simulink model "DoorLockCompositional"  (R2017b)
settings: Solver=FixedStepDiscrete  StartTime=0.0  StopTime=10.0  FixedStep=0.2  RelTol=1e-3
model workspace (MAT data in the model file):
  ContractValidatorBlocksMap = containers.Map
  ContractValidatorBlocksMap.serialization.keys = {'DoorLockCompositional/Lock/ControlSpec/validator', 'DoorLockCompositional/Lock/Keypad/CodeSpec/validator', 'DoorLockCompositional/Lock/KeypadSpec/validator', 'DoorLockCompositional/LockSpec/validator'}
  ContractValidatorBlocksMap.serialization.values{1}.block = 'DoorLockCompositional/Lock/ControlSpec/validator'
  ContractValidatorBlocksMap.serialization.values{1}.assumePorts = 0
  ContractValidatorBlocksMap.serialization.values{1}.guaranteePorts = 1
  ContractValidatorBlocksMap.serialization.values{1}.modeBlocksPorts = 0
  ContractValidatorBlocksMap.serialization.values{1}.portHandles.Inport = 2581.00549316
  ContractValidatorBlocksMap.serialization.values{1}.portHandles.Outport = 2582.00585938
  ContractValidatorBlocksMap.serialization.values{1}.portHandles.Enable = []
  ContractValidatorBlocksMap.serialization.values{1}.portHandles.Trigger = []
  ContractValidatorBlocksMap.serialization.values{1}.portHandles.State = []
  ContractValidatorBlocksMap.serialization.values{1}.portHandles.LConn = []
  ContractValidatorBlocksMap.serialization.values{1}.portHandles.RConn = []
  ContractValidatorBlocksMap.serialization.values{1}.portHandles.Ifaction = []
  ContractValidatorBlocksMap.serialization.values{1}.portHandles.Reset = []
  ContractValidatorBlocksMap.serialization.values{1}.portConnectivity(1).Type = '1'
  ContractValidatorBlocksMap.serialization.values{1}.portConnectivity(1).Position = [370 85]
  ContractValidatorBlocksMap.serialization.values{1}.portConnectivity(1).SrcBlock = 1865.00183105
  ContractValidatorBlocksMap.serialization.values{1}.portConnectivity(1).SrcPort = 0
  ContractValidatorBlocksMap.serialization.values{1}.portConnectivity(1).DstBlock = []
  ContractValidatorBlocksMap.serialization.values{1}.portConnectivity(1).DstPort = []
  ContractValidatorBlocksMap.serialization.values{1}.portConnectivity(2).Type = '1'
  ContractValidatorBlocksMap.serialization.values{1}.portConnectivity(2).Position = [500 85]
  ContractValidatorBlocksMap.serialization.values{1}.portConnectivity(2).SrcBlock = []
  ContractValidatorBlocksMap.serialization.values{1}.portConnectivity(2).SrcPort = []
  ContractValidatorBlocksMap.serialization.values{1}.portConnectivity(2).DstBlock = 1886.00170898
  ContractValidatorBlocksMap.serialization.values{1}.portConnectivity(2).DstPort = 0
  ContractValidatorBlocksMap.serialization.values{2}.block = 'DoorLockCompositional/Lock/Keypad/CodeSpec/validator'
  ContractValidatorBlocksMap.serialization.values{2}.assumePorts = 1
  ContractValidatorBlocksMap.serialization.values{2}.guaranteePorts = 1
  ContractValidatorBlocksMap.serialization.values{2}.modeBlocksPorts = 0
  ContractValidatorBlocksMap.serialization.values{2}.portHandles.Inport = [2578.0057373 2579.00598145]
  ContractValidatorBlocksMap.serialization.values{2}.portHandles.Outport = 2580.00585938
  ContractValidatorBlocksMap.serialization.values{2}.portHandles.Enable = []
  ContractValidatorBlocksMap.serialization.values{2}.portHandles.Trigger = []
  ContractValidatorBlocksMap.serialization.values{2}.portHandles.State = []
  ContractValidatorBlocksMap.serialization.values{2}.portHandles.LConn = []
  ContractValidatorBlocksMap.serialization.values{2}.portHandles.RConn = []
  ContractValidatorBlocksMap.serialization.values{2}.portHandles.Ifaction = []
  ContractValidatorBlocksMap.serialization.values{2}.portHandles.Reset = []
  ContractValidatorBlocksMap.serialization.values{2}.portConnectivity(1).Type = '1'
  ContractValidatorBlocksMap.serialization.values{2}.portConnectivity(1).Position = [385 50]
  ContractValidatorBlocksMap.serialization.values{2}.portConnectivity(1).SrcBlock = 1945.00256348
  ContractValidatorBlocksMap.serialization.values{2}.portConnectivity(1).SrcPort = 0
  ContractValidatorBlocksMap.serialization.values{2}.portConnectivity(1).DstBlock = []
  ContractValidatorBlocksMap.serialization.values{2}.portConnectivity(1).DstPort = []
  ContractValidatorBlocksMap.serialization.values{2}.portConnectivity(2).Type = '2'
  ContractValidatorBlocksMap.serialization.values{2}.portConnectivity(2).Position = [385 100]
  ContractValidatorBlocksMap.serialization.values{2}.portConnectivity(2).SrcBlock = 1959.00610352
  ContractValidatorBlocksMap.serialization.values{2}.portConnectivity(2).SrcPort = 0
  ContractValidatorBlocksMap.serialization.values{2}.portConnectivity(2).DstBlock = []
  ContractValidatorBlocksMap.serialization.values{2}.portConnectivity(2).DstPort = []
  ContractValidatorBlocksMap.serialization.values{2}.portConnectivity(3).Type = '1'
  ContractValidatorBlocksMap.serialization.values{2}.portConnectivity(3).Position = [475 75]
  ContractValidatorBlocksMap.serialization.values{2}.portConnectivity(3).SrcBlock = []
  ContractValidatorBlocksMap.serialization.values{2}.portConnectivity(3).SrcPort = []
  ContractValidatorBlocksMap.serialization.values{2}.portConnectivity(3).DstBlock = 1975.00280762
  ContractValidatorBlocksMap.serialization.values{2}.portConnectivity(3).DstPort = 0
  ContractValidatorBlocksMap.serialization.values{3}.block = 'DoorLockCompositional/Lock/KeypadSpec/validator'
  ContractValidatorBlocksMap.serialization.values{3}.assumePorts = 1
  ContractValidatorBlocksMap.serialization.values{3}.guaranteePorts = 5
  ContractValidatorBlocksMap.serialization.values{3}.modeBlocksPorts = 0
  ContractValidatorBlocksMap.serialization.values{3}.portHandles.Inport = [2571.00695801 2572.00598145 2573.0057373 2574.0057373 2575.0057373 2576.0057373]
  ContractValidatorBlocksMap.serialization.values{3}.portHandles.Outport = 2577.0057373
  ContractValidatorBlocksMap.serialization.values{3}.portHandles.Enable = []
  ContractValidatorBlocksMap.serialization.values{3}.portHandles.Trigger = []
  ContractValidatorBlocksMap.serialization.values{3}.portHandles.State = []
  ContractValidatorBlocksMap.serialization.values{3}.portHandles.LConn = []
  ContractValidatorBlocksMap.serialization.values{3}.portHandles.RConn = []
  ContractValidatorBlocksMap.serialization.values{3}.portHandles.Ifaction = []
  ContractValidatorBlocksMap.serialization.values{3}.portHandles.Reset = []
  ContractValidatorBlocksMap.serialization.values{3}.portConnectivity(1).Type = '1'
  ContractValidatorBlocksMap.serialization.values{3}.portConnectivity(1).Position = [365 -125]
  ContractValidatorBlocksMap.serialization.values{3}.portConnectivity(1).SrcBlock = 2195.00146484
  ContractValidatorBlocksMap.serialization.values{3}.portConnectivity(1).SrcPort = 0
  ContractValidatorBlocksMap.serialization.values{3}.portConnectivity(1).DstBlock = []
  ContractValidatorBlocksMap.serialization.values{3}.portConnectivity(1).DstPort = []
  ContractValidatorBlocksMap.serialization.values{3}.portConnectivity(2).Type = '2'
  ContractValidatorBlocksMap.serialization.values{3}.portConnectivity(2).Position = [365 -40]
  ContractValidatorBlocksMap.serialization.values{3}.portConnectivity(2).SrcBlock = 2229.00427246
  ContractValidatorBlocksMap.serialization.values{3}.portConnectivity(2).SrcPort = 0
  ContractValidatorBlocksMap.serialization.values{3}.portConnectivity(2).DstBlock = []
  ContractValidatorBlocksMap.serialization.values{3}.portConnectivity(2).DstPort = []
  ContractValidatorBlocksMap.serialization.values{3}.portConnectivity(3).Type = '3'
  ContractValidatorBlocksMap.serialization.values{3}.portConnectivity(3).Position = [365 45]
  ContractValidatorBlocksMap.serialization.values{3}.portConnectivity(3).SrcBlock = 2207.00341797
  ContractValidatorBlocksMap.serialization.values{3}.portConnectivity(3).SrcPort = 0
  ContractValidatorBlocksMap.serialization.values{3}.portConnectivity(3).DstBlock = []
  ContractValidatorBlocksMap.serialization.values{3}.portConnectivity(3).DstPort = []
  ContractValidatorBlocksMap.serialization.values{3}.portConnectivity(4).Type = '4'
  ContractValidatorBlocksMap.serialization.values{3}.portConnectivity(4).Position = [365 130]
  ContractValidatorBlocksMap.serialization.values{3}.portConnectivity(4).SrcBlock = 2257.01599121
  ContractValidatorBlocksMap.serialization.values{3}.portConnectivity(4).SrcPort = 0
  ContractValidatorBlocksMap.serialization.values{3}.portConnectivity(4).DstBlock = []
  ContractValidatorBlocksMap.serialization.values{3}.portConnectivity(4).DstPort = []
  ContractValidatorBlocksMap.serialization.values{3}.portConnectivity(5).Type = '5'
  ContractValidatorBlocksMap.serialization.values{3}.portConnectivity(5).Position = [365 215]
  ContractValidatorBlocksMap.serialization.values{3}.portConnectivity(5).SrcBlock = 2223.0057373
  ContractValidatorBlocksMap.serialization.values{3}.portConnectivity(5).SrcPort = 0
  ContractValidatorBlocksMap.serialization.values{3}.portConnectivity(5).DstBlock = []
  ContractValidatorBlocksMap.serialization.values{3}.portConnectivity(5).DstPort = []
  ContractValidatorBlocksMap.serialization.values{3}.portConnectivity(6).Type = '6'
  ContractValidatorBlocksMap.serialization.values{3}.portConnectivity(6).Position = [365 300]
  ContractValidatorBlocksMap.serialization.values{3}.portConnectivity(6).SrcBlock = 2247.00708008
  ContractValidatorBlocksMap.serialization.values{3}.portConnectivity(6).SrcPort = 0
  ContractValidatorBlocksMap.serialization.values{3}.portConnectivity(6).DstBlock = []
  ContractValidatorBlocksMap.serialization.values{3}.portConnectivity(6).DstPort = []
  ContractValidatorBlocksMap.serialization.values{3}.portConnectivity(7).Type = '1'
  ContractValidatorBlocksMap.serialization.values{3}.portConnectivity(7).Position = [500 90]
  ContractValidatorBlocksMap.serialization.values{3}.portConnectivity(7).SrcBlock = []
  ContractValidatorBlocksMap.serialization.values{3}.portConnectivity(7).SrcPort = []
  ContractValidatorBlocksMap.serialization.values{3}.portConnectivity(7).DstBlock = [2282.00183105 2194.00244141]
  ContractValidatorBlocksMap.serialization.values{3}.portConnectivity(7).DstPort = [0 0]
  ContractValidatorBlocksMap.serialization.values{4}.block = 'DoorLockCompositional/LockSpec/validator'
  ContractValidatorBlocksMap.serialization.values{4}.assumePorts = 1
  ContractValidatorBlocksMap.serialization.values{4}.guaranteePorts = 2
  ContractValidatorBlocksMap.serialization.values{4}.modeBlocksPorts = 0
  ContractValidatorBlocksMap.serialization.values{4}.portHandles.Inport = [2583.00549316 2584.00549316 2585.00585938]
  ContractValidatorBlocksMap.serialization.values{4}.portHandles.Outport = 2586.00549316
  ContractValidatorBlocksMap.serialization.values{4}.portHandles.Enable = []
  ContractValidatorBlocksMap.serialization.values{4}.portHandles.Trigger = []
  ContractValidatorBlocksMap.serialization.values{4}.portHandles.State = []
  ContractValidatorBlocksMap.serialization.values{4}.portHandles.LConn = []
  ContractValidatorBlocksMap.serialization.values{4}.portHandles.RConn = []
  ContractValidatorBlocksMap.serialization.values{4}.portHandles.Ifaction = []
  ContractValidatorBlocksMap.serialization.values{4}.portHandles.Reset = []
  ContractValidatorBlocksMap.serialization.values{4}.portConnectivity(1).Type = '1'
  ContractValidatorBlocksMap.serialization.values{4}.portConnectivity(1).Position = [445 -95]
  ContractValidatorBlocksMap.serialization.values{4}.portConnectivity(1).SrcBlock = 2413.00170898
  ContractValidatorBlocksMap.serialization.values{4}.portConnectivity(1).SrcPort = 0
  ContractValidatorBlocksMap.serialization.values{4}.portConnectivity(1).DstBlock = []
  ContractValidatorBlocksMap.serialization.values{4}.portConnectivity(1).DstPort = []
  ContractValidatorBlocksMap.serialization.values{4}.portConnectivity(2).Type = '2'
  ContractValidatorBlocksMap.serialization.values{4}.portConnectivity(2).Position = [445 75]
  ContractValidatorBlocksMap.serialization.values{4}.portConnectivity(2).SrcBlock = 2425.00341797
  ContractValidatorBlocksMap.serialization.values{4}.portConnectivity(2).SrcPort = 0
  ContractValidatorBlocksMap.serialization.values{4}.portConnectivity(2).DstBlock = []
  ContractValidatorBlocksMap.serialization.values{4}.portConnectivity(2).DstPort = []
  ContractValidatorBlocksMap.serialization.values{4}.portConnectivity(3).Type = '3'
  ContractValidatorBlocksMap.serialization.values{4}.portConnectivity(3).Position = [445 245]
  ContractValidatorBlocksMap.serialization.values{4}.portConnectivity(3).SrcBlock = 2431.00341797
  ContractValidatorBlocksMap.serialization.values{4}.portConnectivity(3).SrcPort = 0
  ContractValidatorBlocksMap.serialization.values{4}.portConnectivity(3).DstBlock = []
  ContractValidatorBlocksMap.serialization.values{4}.portConnectivity(3).DstPort = []
  ContractValidatorBlocksMap.serialization.values{4}.portConnectivity(4).Type = '1'
  ContractValidatorBlocksMap.serialization.values{4}.portConnectivity(4).Position = [580 75]
  ContractValidatorBlocksMap.serialization.values{4}.portConnectivity(4).SrcBlock = []
  ContractValidatorBlocksMap.serialization.values{4}.portConnectivity(4).SrcPort = []
  ContractValidatorBlocksMap.serialization.values{4}.portConnectivity(4).DstBlock = [2539.00231934 2411.00268555]
  ContractValidatorBlocksMap.serialization.values{4}.portConnectivity(4).DstPort = [0 0]
  ContractValidatorBlocksMap.serialization.uniformity = 0
  ContractValidatorBlocksMap.serialization.keyType = 'char'
  ContractValidatorBlocksMap.serialization.valueType = 'any'
undefined symbols (not defined in the file): contractAfterSimulation, ContractAssumeBlock, contractBeforeSimulation, ContractBlock, ContractGuaranteeBlock, ContractValidatorBlock, saveValidatorParameters
libraries: simulink x17, Kind x15
settings Model: Creator=mahgoubyahia  LastModifiedBy=hbourbou
settings OptimizationCC: LifeSpan=inf
settings DebuggingCC: SFExecutionAtInitializationDiag=none
settings HardwareCC: ProdBitPerSizeT=32  ProdBitPerPtrDiffT=32  ProdWordSize=32  ProdHWDeviceType=Specified
settings CodeAppCC: StateflowObjectComments=on

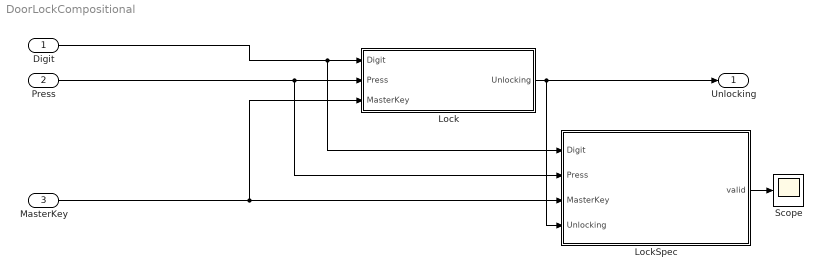
== system DoorLockCompositional ==
  Digit : Inport  OutDataTypeStr=int8
  Press : Inport  Port=2  OutDataTypeStr=boolean
  MasterKey : Inport  Port=3  OutDataTypeStr=boolean
  Lock : Subsystem
  LockSpec : Subsystem  mask(ContractBlock){ContractBlockType=ContractBlock}
      mask DialogControl DescTextVar Prompt: Contract block
      mask Display:
      | text(0.5, 0.5, '{\bf\fontsize{20}Contract}', 'hor', 'center', 'texmode','on');
      | blocks = find_system(gcb, 'LookUnderMasks','all', 'SearchDepth',1,'BlockType','Inport');
      | for i = 1 : length(blocks)
      |     blockName = get_param(blocks(i), 'Name');
      |     [path, blockName] = fileparts(char(blockName));
      |     port_label('input', i, blockName);
      | end
      | 
      | blocks = find_system(gcb, 'LookUnderMasks','all', 'SearchDepth',1,'BlockType','Outport');
      | for i = 1 : length(blocks)
      |     blockName = get_param(blocks(i), 'Name');
      |     [path, blockName] = fileparts(char(blockName));
      |     port_label('output', i, blockName);
      | end
  Scope : Scope
  Unlocking : Outport  OutDataTypeStr=boolean
  wires:
  Digit/1 -> LockSpec/1(Digit), Lock/1(Digit)
  Press/1 -> LockSpec/2(Press), Lock/2(Press)
  MasterKey/1 -> Lock/3(MasterKey), LockSpec/3(MasterKey)
  Lock/1(Unlocking) -> LockSpec/4(Unlocking), Unlocking/1
  LockSpec/1(valid) -> Scope/1

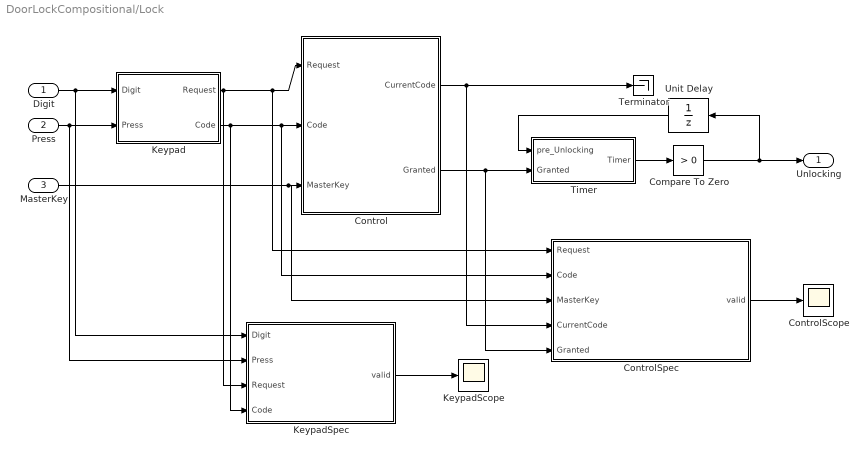
== system DoorLockCompositional/Lock ==
  Digit : Inport  OutDataTypeStr=int8
  Press : Inport  Port=2  OutDataTypeStr=boolean
  MasterKey : Inport  Port=3  OutDataTypeStr=boolean
  Compare To Zero : simulink/Logic and Bit Operations/Compare To Zero  relop=>  OutDataTypeStr=boolean
  Control : Subsystem
  ControlScope : Scope
  ControlSpec : Subsystem  AncestorBlock=Kind/contract  mask(ContractBlock){ContractBlockType=ContractBlock}
      mask init:
      | set_param(gcb, 'LinkStatus', 'inactive');
      mask DialogControl DescTextVar Prompt: Contract block
      mask Display:
      | text(0.5, 0.5, '{\bf\fontsize{20}Contract}', 'hor', 'center', 'texmode','on');
      | blocks = find_system(gcb, 'LookUnderMasks','all', 'SearchDepth',1,'BlockType','Inport');
      | for i = 1 : length(blocks)
      |     blockName = get_param(blocks(i), 'Name');
      |     [path, blockName] = fileparts(char(blockName));
      |     port_label('input', i, blockName);
      | end
      | 
      | blocks = find_system(gcb, 'LookUnderMasks','all', 'SearchDepth',1,'BlockType','Outport');
      | for i = 1 : length(blocks)
      |     blockName = get_param(blocks(i), 'Name');
      |     [path, blockName] = fileparts(char(blockName));
      |     port_label('output', i, blockName);
      | end
  Keypad : Subsystem
  KeypadScope : Scope
  KeypadSpec : Subsystem  mask(ContractBlock){ContractBlockType=ContractBlock}
      mask init:
      | set_param(gcb, 'LinkStatus', 'none');
      mask DialogControl DescTextVar Prompt: Contract block
      mask Display:
      | text(0.5, 0.5, '{\bf\fontsize{20}Contract}', 'hor', 'center', 'texmode','on');
      | blocks = find_system(gcb, 'LookUnderMasks','all', 'SearchDepth',1,'BlockType','Inport');
      | for i = 1 : length(blocks)
      |     blockName = get_param(blocks(i), 'Name');
      |     [path, blockName] = fileparts(char(blockName));
      |     port_label('input', i, blockName);
      | end
      | 
      | blocks = find_system(gcb, 'LookUnderMasks','all', 'SearchDepth',1,'BlockType','Outport');
      | for i = 1 : length(blocks)
      |     blockName = get_param(blocks(i), 'Name');
      |     [path, blockName] = fileparts(char(blockName));
      |     port_label('output', i, blockName);
      | end
  Terminator : Terminator
  Timer : Subsystem
  Unit Delay : UnitDelay  SampleTime=-1
  Unlocking : Outport  OutDataTypeStr=boolean
  wires:
  Control/1(CurrentCode) -> ControlSpec/4(CurrentCode), Terminator/1
  Keypad/2(Code) -> KeypadSpec/4(Code), Control/2(Code), ControlSpec/2(Code)
  Keypad/1(Request) -> KeypadSpec/3(Request), Control/1(Request), ControlSpec/1(Request)
  MasterKey/1 -> ControlSpec/3(MasterKey), Control/3(MasterKey)
  Timer/1(Timer) -> Compare To Zero/1
  Compare To Zero/1 -> Unlocking/1, Unit Delay/1
  Press/1 -> KeypadSpec/2(Press), Keypad/2(Press)
  Digit/1 -> KeypadSpec/1(Digit), Keypad/1(Digit)
  Control/2(Granted) -> ControlSpec/5(Granted), Timer/2(Granted)
  ControlSpec/1(valid) -> ControlScope/1
  KeypadSpec/1(valid) -> KeypadScope/1
  Unit Delay/1 -> Timer/1(pre_Unlocking)

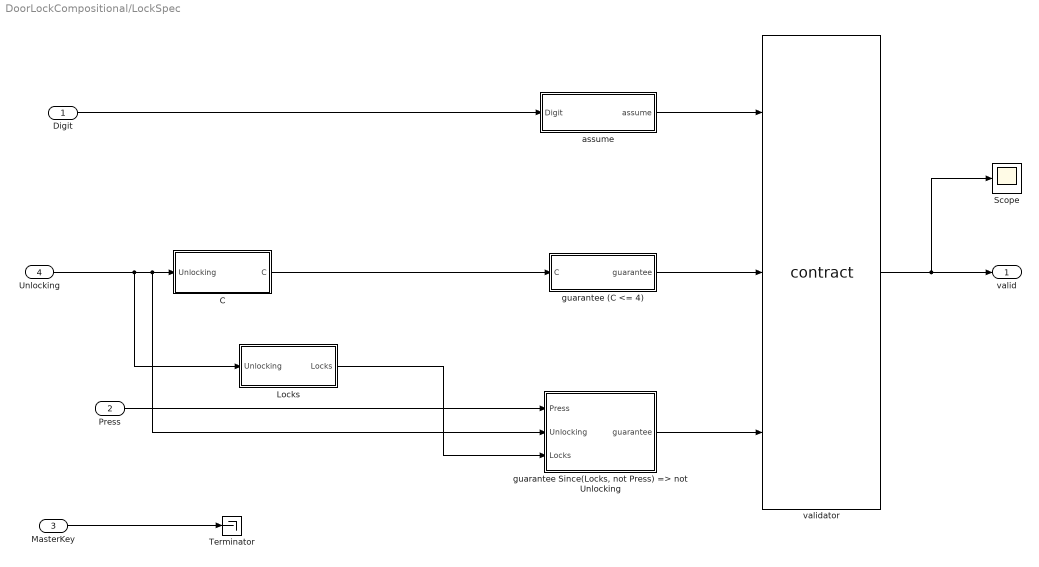
== system DoorLockCompositional/LockSpec ==
  Digit : Inport
  Press : Inport  Port=2  OutDataTypeStr=boolean
  MasterKey : Inport  Port=3  OutDataTypeStr=boolean
  Unlocking : Inport  Port=4  OutDataTypeStr=boolean
  C : Subsystem
  Locks : Subsystem
  Scope : Scope
  Terminator : Terminator
  assume : Subsystem  AncestorBlock=Kind/assume  mask(ContractAssumeBlock){ContractBlockType=ContractAssumeBlock}
      mask DialogControl DescTextVar Prompt: Assume block
  guarantee (C <= 4) : Subsystem  AncestorBlock=Kind/guarantee  mask(ContractGuaranteeBlock){ContractBlockType=ContractGuaranteeBlock}
      mask DialogControl DescTextVar Prompt: Guarantee block
  "guarantee Since(Locks, not Press) => not Unlocking" : Subsystem  AncestorBlock=Kind/guarantee  mask(ContractGuaranteeBlock){ContractBlockType=ContractGuaranteeBlock}
      mask DialogControl DescTextVar Prompt: Guarantee block
  validator : M-S-Function  LoadFcn=saveValidatorParameters(gcb);  InitFcn=contractBeforeSimulation();  StopFcn=contractAfterSimulation();  FunctionName=contract  mask(ContractValidatorBlock){assumePorts=1, guaranteePorts=2, modePorts=0, ContractBlockType=ContractValidatorBlock, createInportsCheckbox=off}
      mask prompts: assumePorts "Assume ports     :"; guaranteePorts "Guarantee ports :"; modePorts "Mode ports        :"; createInportsCheckbox "Create inports and connect them automatically"
      mask init:
      | set_param(gcb,'LinkStatus','none');
      | contract_callback('inputs_callback',gcb);
      mask DialogControl DescTextVar Prompt: The validator block implements the following logic: <br> <br> <b>Sofar</b>(assume<sub>1</sub> <b>&#8743;</b> assume<sub>2</sub> <b>&#8743;</b> ... assume<sub>k</sub>) <b>&rarr;</b> (guarantee<sub>1</sub> <b>&#8743;</b> guarantee<sub>2</sub> <b>&#8743;</b> ... guarantee<sub>m</sub> <b>&#8743;</b>  mode<sub>1</sub> <b>&#8743;</b> mode<sub>2</sub> <b>&#8743;</b> ... <b>&#8743;</b> mode<sub>n</sub> )<br> where mode<sub>i</sub> = require<sub>i</sub> <b>&rarr;</b> ensure<sub>i</sub>
      mask Display:
      | color('black');
      | port_label('input',1,'assume');
      | port_label('input',2,'guarantee');
      | port_label('input',3,'guarantee');
      | port_label('output',1,'valid');
  valid : Outport
  wires:
  validator/1 -> Scope/1, valid/1
  assume/1(assume) -> validator/1
  guarantee (C <= 4)/1(guarantee) -> validator/2
  "guarantee Since(Locks, not Press) => not Unlocking"/1(guarantee) -> validator/3
  Digit/1 -> assume/1(Digit)
  Press/1 -> "guarantee Since(Locks, not Press) => not Unlocking"/1(Press)
  Unlocking/1 -> Locks/1(Unlocking), "guarantee Since(Locks, not Press) => not Unlocking"/2(Unlocking), C/1(Unlocking)
  C/1(C) -> guarantee (C <= 4)/1(C)
  MasterKey/1 -> Terminator/1
  Locks/1(Locks) -> "guarantee Since(Locks, not Press) => not Unlocking"/3(Locks)

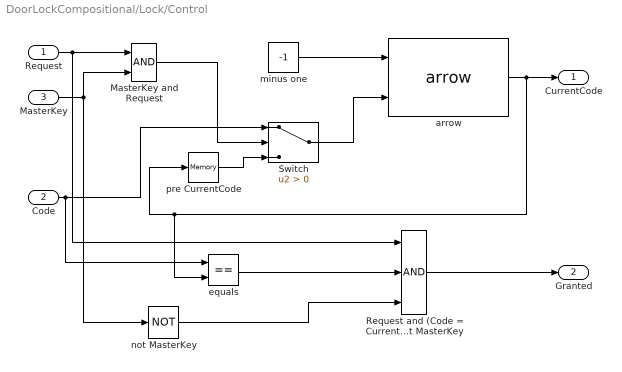
== system DoorLockCompositional/Lock/Control ==
  Request : Inport  OutDataTypeStr=boolean
  Code : Inport  Port=2  OutDataTypeStr=int32
  MasterKey : Inport  Port=3  OutDataTypeStr=boolean
  MasterKey and Request : Logic  IconShape=distinctive  AllPortsSameDT=off  OutDataTypeStr=boolean
  Request and (Code = CurrentCode) and not MasterKey : Logic  Inputs=3  IconShape=distinctive  AllPortsSameDT=off  OutDataTypeStr=boolean
  Switch : Switch  Criteria=u2 > Threshold
  arrow : Kind/arrow  LustreOperatorBlock=ArrowOperator
  equals : RelationalOperator  Operator===  OutDataTypeStr=boolean  RndMeth=Nearest
  minus one : Constant  Value=-1  OutDataTypeStr=int32
  "not MasterKey " : Logic  Operator=NOT  IconShape=distinctive  AllPortsSameDT=off  OutDataTypeStr=boolean
  pre CurrentCode : Memory
  CurrentCode : Outport  OutDataTypeStr=int32
  Granted : Outport  Port=2  OutDataTypeStr=boolean
  wires:
  arrow/1 -> equals/2, pre CurrentCode/1, CurrentCode/1
  minus one/1 -> arrow/1
  Request/1 -> MasterKey and Request/1, Request and (Code = CurrentCode) and not MasterKey/1
  MasterKey/1 -> "not MasterKey "/1, MasterKey and Request/2
  MasterKey and Request/1 -> Switch/2
  Code/1 -> equals/1, Switch/1
  pre CurrentCode/1 -> Switch/3
  Switch/1 -> arrow/2
  equals/1 -> Request and (Code = CurrentCode) and not MasterKey/2
  "not MasterKey "/1 -> Request and (Code = CurrentCode) and not MasterKey/3
  Request and (Code = CurrentCode) and not MasterKey/1 -> Granted/1

== system DoorLockCompositional/Lock/ControlSpec ==
  Request : Inport  OutDataTypeStr=boolean
  Code : Inport  Port=2  OutDataTypeStr=int32
  MasterKey : Inport  Port=3  OutDataTypeStr=boolean
  CurrentCode : Inport  Port=4  OutDataTypeStr=int32
  Granted : Inport  Port=5  OutDataTypeStr=boolean
  guarantee true : Subsystem  mask(ContractGuaranteeBlock){ContractBlockType=ContractGuaranteeBlock}
      mask init:
      | set_param(gcb, 'LinkStatus', 'none');
      mask DialogControl DescTextVar Prompt: Guarantee block
  validator : M-S-Function  LoadFcn=saveValidatorParameters(gcb);  InitFcn=contractBeforeSimulation();  StopFcn=contractAfterSimulation();  FunctionName=contract  mask(ContractValidatorBlock){assumePorts=0, guaranteePorts=1, modePorts=0, ContractBlockType=ContractValidatorBlock, createInportsCheckbox=off}
      mask prompts: assumePorts "Assume ports     :"; guaranteePorts "Guarantee ports :"; modePorts "Mode ports        :"; createInportsCheckbox "Create inports and connect them automatically"
      mask init:
      | set_param(gcb,'LinkStatus','none');
      | contract_callback('inputs_callback',gcb);
      mask DialogControl DescTextVar Prompt: The validator block implements the following logic: <br> <br> <b>Sofar</b>(assume<sub>1</sub> <b>&#8743;</b> assume<sub>2</sub> <b>&#8743;</b> ... assume<sub>k</sub>) <b>&rarr;</b> (guarantee<sub>1</sub> <b>&#8743;</b> guarantee<sub>2</sub> <b>&#8743;</b> ... guarantee<sub>m</sub> <b>&#8743;</b>  mode<sub>1</sub> <b>&#8743;</b> mode<sub>2</sub> <b>&#8743;</b> ... <b>&#8743;</b> mode<sub>n</sub> )<br> where mode<sub>i</sub> = require<sub>i</sub> <b>&rarr;</b> ensure<sub>i</sub>
      mask Display:
      | color('black');
      | port_label('input',1,'guarantee');
      | port_label('output',1,'valid');
  valid : Outport
  wires:
  validator/1 -> valid/1
  guarantee true/1(guarantee) -> validator/1
  Request/1 -> guarantee true/1(Request)
  Code/1 -> guarantee true/2(Code)
  MasterKey/1 -> guarantee true/3(MasterKey)
  CurrentCode/1 -> guarantee true/4(CurrentCode)
  Granted/1 -> guarantee true/5(Granted)

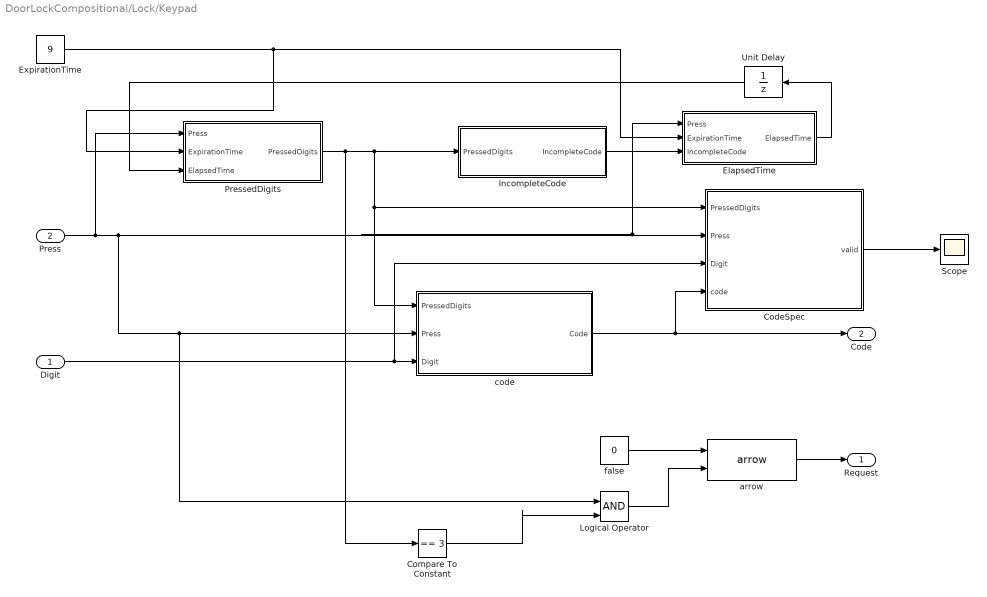
== system DoorLockCompositional/Lock/Keypad ==
  Digit : Inport
  Press : Inport  Port=2  OutDataTypeStr=boolean
  CodeSpec : Subsystem  mask(ContractBlock){ContractBlockType=ContractBlock}
      mask init:
      | set_param(gcb, 'LinkStatus', 'none');
      settings: CopyFcn=set_param(gcb, 'LinkStatus', 'none');
      mask DialogControl DescTextVar Prompt: Contract block
      mask Display:
      | text(0.5, 0.5, '{\bf\fontsize{20}Contract}', 'hor', 'center', 'texmode','on');
      | blocks = find_system(gcb, 'LookUnderMasks','all', 'SearchDepth',1,'BlockType','Inport');
      | for i = 1 : length(blocks)
      |     blockName = get_param(blocks(i), 'Name');
      |     [path, blockName] = fileparts(char(blockName));
      |     port_label('input', i, blockName);
      | end
      | 
      | blocks = find_system(gcb, 'LookUnderMasks','all', 'SearchDepth',1,'BlockType','Outport');
      | for i = 1 : length(blocks)
      |     blockName = get_param(blocks(i), 'Name');
      |     [path, blockName] = fileparts(char(blockName));
      |     port_label('output', i, blockName);
      | end
  Compare To Constant : simulink/Logic and Bit Operations/Compare To Constant  relop===  const=3  OutDataTypeStr=boolean
  ElapsedTime : Subsystem
  ExpirationTime : Constant  Value=9  OutDataTypeStr=int32
  IncompleteCode : Subsystem
  Logical Operator : Logic  IconShape=distinctive  AllPortsSameDT=off  OutDataTypeStr=boolean
  PressedDigits : Subsystem
  Scope : Scope
  Unit Delay : UnitDelay  SampleTime=-1
  arrow : Kind/arrow  LustreOperatorBlock=ArrowOperator
  code : Subsystem
  false : Constant  Value=0  OutDataTypeStr=boolean
  Request : Outport  OutDataTypeStr=boolean
  Code : Outport  Port=2  OutDataTypeStr=int32
  wires:
  PressedDigits/1(PressedDigits) -> Compare To Constant/1, code/1(PressedDigits), CodeSpec/1(PressedDigits), IncompleteCode/1(PressedDigits)
  Press/1 -> PressedDigits/1(Press), Logical Operator/1, code/2(Press), CodeSpec/2(Press), ElapsedTime/1(Press)
  ExpirationTime/1 -> ElapsedTime/2(ExpirationTime), PressedDigits/2(ExpirationTime)
  IncompleteCode/1(IncompleteCode) -> ElapsedTime/3(IncompleteCode)
  ElapsedTime/1(ElapsedTime) -> Unit Delay/1
  Digit/1 -> CodeSpec/3(Digit), code/3(Digit)
  code/1(Code) -> CodeSpec/4(code), Code/1
  arrow/1 -> Request/1
  false/1 -> arrow/1
  Logical Operator/1 -> arrow/2
  Compare To Constant/1 -> Logical Operator/2
  CodeSpec/1(valid) -> Scope/1
  Unit Delay/1 -> PressedDigits/3(ElapsedTime)

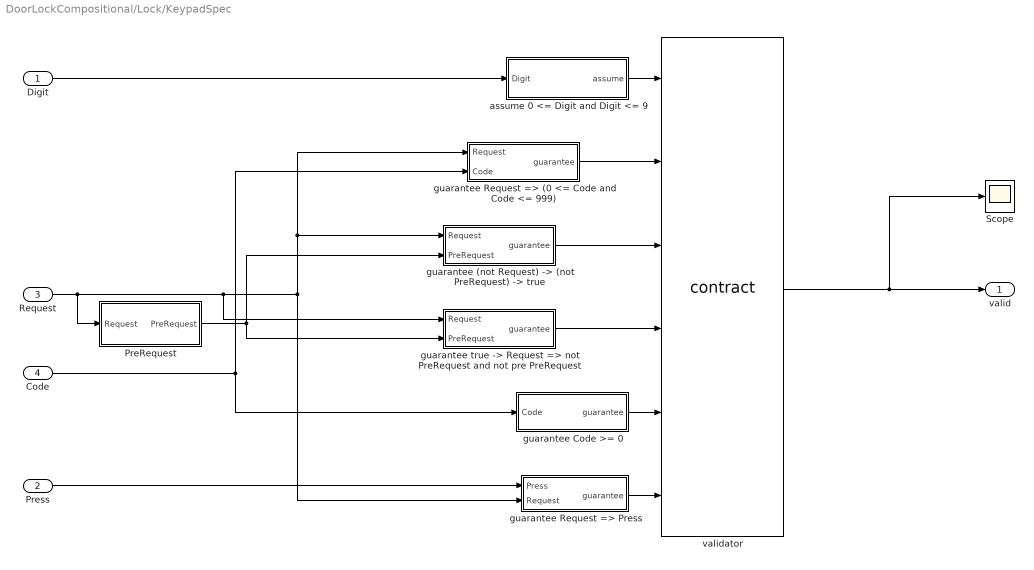
== system DoorLockCompositional/Lock/KeypadSpec ==
  Digit : Inport
  Press : Inport  Port=2  OutDataTypeStr=boolean
  Request : Inport  Port=3  OutDataTypeStr=boolean
  Code : Inport  Port=4  OutDataTypeStr=int32
  PreRequest : Subsystem
  Scope : Scope
  assume 0 <= Digit and Digit <= 9 : Subsystem  mask(ContractAssumeBlock){ContractBlockType=ContractAssumeBlock}
      mask init:
      | set_param(gcb, 'LinkStatus', 'none');
      mask DialogControl DescTextVar Prompt: Assume block
  "guarantee (not Request) -> (not PreRequest) -> true" : Subsystem  mask(ContractGuaranteeBlock){ContractBlockType=ContractGuaranteeBlock}
      mask init:
      | set_param(gcb, 'LinkStatus', 'none');
      mask DialogControl DescTextVar Prompt: Guarantee block
  guarantee Code >= 0 : Subsystem  mask(ContractGuaranteeBlock){ContractBlockType=ContractGuaranteeBlock}
      mask init:
      | set_param(gcb, 'LinkStatus', 'none');
      mask DialogControl DescTextVar Prompt: Guarantee block
  guarantee Request => (0 <= Code and Code <= 999) : Subsystem  mask(ContractGuaranteeBlock){ContractBlockType=ContractGuaranteeBlock}
      mask init:
      | set_param(gcb, 'LinkStatus', 'none');
      mask DialogControl DescTextVar Prompt: Guarantee block
  guarantee Request => Press : Subsystem  mask(ContractGuaranteeBlock){ContractBlockType=ContractGuaranteeBlock}
      mask init:
      | set_param(gcb, 'LinkStatus', 'none');
      mask DialogControl DescTextVar Prompt: Guarantee block
  "guarantee true -> Request => not PreRequest and not pre PreRequest" : Subsystem  mask(ContractGuaranteeBlock){ContractBlockType=ContractGuaranteeBlock}
      mask init:
      | set_param(gcb, 'LinkStatus', 'none');
      mask DialogControl DescTextVar Prompt: Guarantee block
  validator : M-S-Function  LoadFcn=saveValidatorParameters(gcb);  InitFcn=contractBeforeSimulation();  StopFcn=contractAfterSimulation();  FunctionName=contract  mask(ContractValidatorBlock){assumePorts=1, guaranteePorts=5, modePorts=0, ContractBlockType=ContractValidatorBlock, createInportsCheckbox=off}
      mask prompts: assumePorts "Assume ports     :"; guaranteePorts "Guarantee ports :"; modePorts "Mode ports        :"; createInportsCheckbox "Create inports and connect them automatically"
      mask init:
      | set_param(gcb,'LinkStatus','none');
      | contract_callback('inputs_callback',gcb);
      mask DialogControl DescTextVar Prompt: The validator block implements the following logic: <br> <br> <b>Sofar</b>(assume<sub>1</sub> <b>&#8743;</b> assume<sub>2</sub> <b>&#8743;</b> ... assume<sub>k</sub>) <b>&rarr;</b> (guarantee<sub>1</sub> <b>&#8743;</b> guarantee<sub>2</sub> <b>&#8743;</b> ... guarantee<sub>m</sub> <b>&#8743;</b>  mode<sub>1</sub> <b>&#8743;</b> mode<sub>2</sub> <b>&#8743;</b> ... <b>&#8743;</b> mode<sub>n</sub> )<br> where mode<sub>i</sub> = require<sub>i</sub> <b>&rarr;</b> ensure<sub>i</sub>
      mask Display:
      | color('black');
      | port_label('input',1,'assume');
      | port_label('input',2,'guarantee');
      | port_label('input',3,'guarantee');
      | port_label('input',4,'guarantee');
      | port_label('input',5,'guarantee');
      | port_label('input',6,'guarantee');
      | port_label('output',1,'valid');
  valid : Outport
  wires:
  validator/1 -> Scope/1, valid/1
  assume 0 <= Digit and Digit <= 9/1(assume) -> validator/1
  guarantee Request => (0 <= Code and Code <= 999)/1(guarantee) -> validator/2
  "guarantee (not Request) -> (not PreRequest) -> true"/1(guarantee) -> validator/3
  guarantee Code >= 0/1(guarantee) -> validator/5
  guarantee Request => Press/1(guarantee) -> validator/6
  Digit/1 -> assume 0 <= Digit and Digit <= 9/1(Digit)
  Press/1 -> guarantee Request => Press/1(Press)
  Request/1 -> PreRequest/1(Request), "guarantee true -> Request => not PreRequest and not pre PreRequest"/1(Request), guarantee Request => Press/2(Request), guarantee Request => (0 <= Code and Code <= 999)/1(Request), "guarantee (not Request) -> (not PreRequest) -> true"/1(Request)
  Code/1 -> guarantee Code >= 0/1(Code), guarantee Request => (0 <= Code and Code <= 999)/2(Code)
  PreRequest/1(PreRequest) -> "guarantee true -> Request => not PreRequest and not pre PreRequest"/2(PreRequest), "guarantee (not Request) -> (not PreRequest) -> true"/2(PreRequest)
  "guarantee true -> Request => not PreRequest and not pre PreRequest"/1(guarantee) -> validator/4

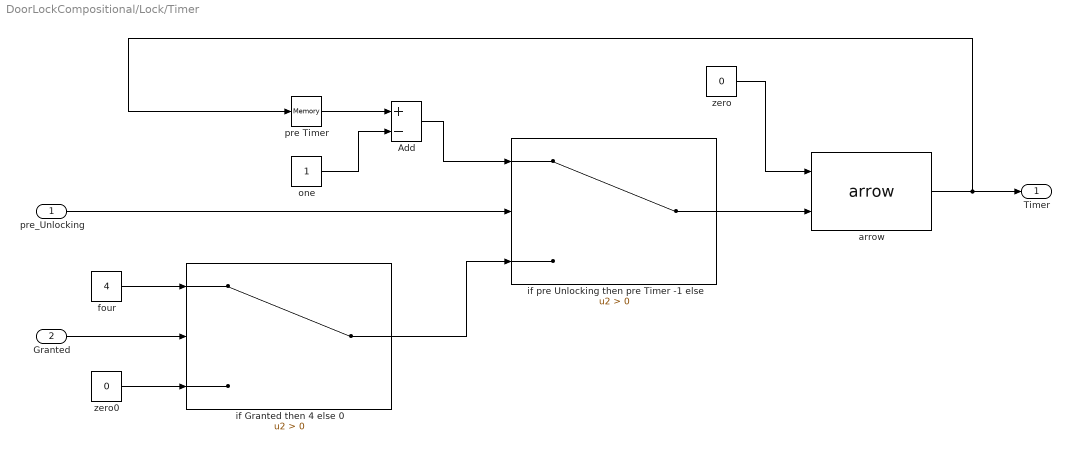
== system DoorLockCompositional/Lock/Timer ==
  pre_Unlocking : Inport  OutDataTypeStr=boolean
  Granted : Inport  Port=2  OutDataTypeStr=boolean
  Add : Sum  Inputs=+-
  arrow : Kind/arrow  LustreOperatorBlock=ArrowOperator
  four : Constant  Value=4  OutDataTypeStr=int32
  if Granted then 4 else 0 : Switch  Criteria=u2 > Threshold
  if pre Unlocking then pre Timer -1 else : Switch  Criteria=u2 > Threshold
  one : Constant  OutDataTypeStr=int32
  pre Timer : Memory
  zero : Constant  Value=0  OutDataTypeStr=int32
  zero0 : Constant  Value=0  OutDataTypeStr=int32
  Timer : Outport
  wires:
  zero/1 -> arrow/1
  arrow/1 -> pre Timer/1, Timer/1
  pre_Unlocking/1 -> if pre Unlocking then pre Timer -1 else/2
  pre Timer/1 -> Add/1
  one/1 -> Add/2
  Add/1 -> if pre Unlocking then pre Timer -1 else/1
  Granted/1 -> if Granted then 4 else 0/2
  four/1 -> if Granted then 4 else 0/1
  zero0/1 -> if Granted then 4 else 0/3
  if Granted then 4 else 0/1 -> if pre Unlocking then pre Timer -1 else/3
  if pre Unlocking then pre Timer -1 else/1 -> arrow/2

== system DoorLockCompositional/LockSpec/C ==
  Unlocking : Inport  OutDataTypeStr=boolean
  Add : Sum
  Switch : Switch  Criteria=u2 > Threshold
  arrow : Kind/arrow  LustreOperatorBlock=ArrowOperator
  one : Constant  OutDataTypeStr=int32
  one1 : Constant  OutDataTypeStr=int32
  pre C : Memory
  zero : Constant  Value=0  OutDataTypeStr=int32
  C : Outport  OutDataTypeStr=int32
  wires:
  Unlocking/1 -> Switch/2
  one/1 -> arrow/1
  one1/1 -> Add/2
  pre C/1 -> Add/1
  Add/1 -> arrow/2
  arrow/1 -> Switch/1
  Switch/1 -> pre C/1, C/1
  zero/1 -> Switch/3

== system DoorLockCompositional/LockSpec/Locks ==
  Unlocking : Inport  OutDataTypeStr=boolean
  and : Logic  IconShape=distinctive  AllPortsSameDT=off  OutDataTypeStr=boolean
  arrow : Kind/arrow  LustreOperatorBlock=ArrowOperator
  false : Constant  Value=0  OutDataTypeStr=boolean
  not Unlocking : Logic  Operator=NOT  IconShape=distinctive  AllPortsSameDT=off  OutDataTypeStr=boolean
  pre Unlocking : Memory
  Locks : Outport  OutDataTypeStr=boolean
  wires:
  false/1 -> arrow/1
  arrow/1 -> Locks/1
  Unlocking/1 -> not Unlocking/1, pre Unlocking/1
  pre Unlocking/1 -> and/1
  not Unlocking/1 -> and/2
  and/1 -> arrow/2

== system DoorLockCompositional/LockSpec/assume ==
  Digit : Inport
  Compare To Constant : simulink/Logic and Bit Operations/Compare To Constant  relop=<=  const=9  OutDataTypeStr=boolean
  Compare To Zero : simulink/Logic and Bit Operations/Compare To Zero  relop=>=  OutDataTypeStr=boolean
  Logical Operator : Logic  IconShape=distinctive  AllPortsSameDT=off  OutDataTypeStr=boolean
  assume : Outport  OutDataTypeStr=boolean
  wires:
  Digit/1 -> Compare To Zero/1, Compare To Constant/1
  Compare To Constant/1 -> Logical Operator/1
  Compare To Zero/1 -> Logical Operator/2
  Logical Operator/1 -> assume/1

== system DoorLockCompositional/LockSpec/guarantee (C <= 4) ==
  C : Inport
  Compare To Constant : simulink/Logic and Bit Operations/Compare To Constant  relop=<=  const=4  OutDataTypeStr=boolean
  guarantee : Outport  OutDataTypeStr=boolean
  wires:
  C/1 -> Compare To Constant/1
  Compare To Constant/1 -> guarantee/1

== system DoorLockCompositional/LockSpec/guarantee Since(Locks, not Press) => not Unlocking ==
  Press : Inport
  Unlocking : Inport  Port=2  OutDataTypeStr=boolean
  Locks : Inport  Port=3  OutDataTypeStr=boolean
  Since : Subsystem
  not Press : Logic  Operator=NOT  IconShape=distinctive  AllPortsSameDT=off  OutDataTypeStr=boolean
  not Since : Logic  Operator=NOT  IconShape=distinctive  AllPortsSameDT=off  OutDataTypeStr=boolean
  not Unlocking : Logic  Operator=NOT  IconShape=distinctive  AllPortsSameDT=off  OutDataTypeStr=boolean
  or : Logic  Operator=OR  IconShape=distinctive  AllPortsSameDT=off  OutDataTypeStr=boolean
  guarantee : Outport  OutDataTypeStr=boolean
  wires:
  not Press/1 -> Since/2(Y)
  Press/1 -> not Press/1
  Locks/1 -> Since/1(X)
  Since/1(SinceXY) -> not Since/1
  not Since/1 -> or/1
  Unlocking/1 -> not Unlocking/1
  not Unlocking/1 -> or/2
  or/1 -> guarantee/1

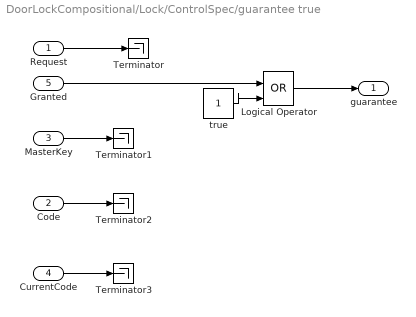
== system DoorLockCompositional/Lock/ControlSpec/guarantee true ==
  Request : Inport
  Code : Inport  Port=2
  MasterKey : Inport  Port=3
  CurrentCode : Inport  Port=4
  Granted : Inport  Port=5
  Logical Operator : Logic  Operator=OR  IconShape=distinctive  AllPortsSameDT=off  OutDataTypeStr=boolean
  Terminator{,1..3} (4 alike) : Terminator
  true : Constant  OutDataTypeStr=boolean
  guarantee : Outport  OutDataTypeStr=boolean
  wires:
  Granted/1 -> Logical Operator/1
  true/1 -> Logical Operator/2
  Logical Operator/1 -> guarantee/1
  Request/1 -> Terminator/1
  MasterKey/1 -> Terminator1/1
  Code/1 -> Terminator2/1
  CurrentCode/1 -> Terminator3/1

== system DoorLockCompositional/Lock/Keypad/CodeSpec ==
  PressedDigits : Inport
  Press : Inport  Port=2
  Digit : Inport  Port=3
  code : Inport  Port=4
  assume 0 <= Digit and Digit <= 9 : Subsystem  mask(ContractAssumeBlock){ContractBlockType=ContractAssumeBlock}
      mask init:
      | set_param(gcb, 'LinkStatus', 'none');
      mask DialogControl DescTextVar Prompt: Assume block
  guarantee code > -5 : Subsystem  mask(ContractGuaranteeBlock){ContractBlockType=ContractGuaranteeBlock}
      mask init:
      | set_param(gcb, 'LinkStatus', 'none');
      mask DialogControl DescTextVar Prompt: Guarantee block
  validator : M-S-Function  LoadFcn=saveValidatorParameters(gcb);  InitFcn=contractBeforeSimulation();  StopFcn=contractAfterSimulation();  FunctionName=contract  mask(ContractValidatorBlock){assumePorts=1, guaranteePorts=1, modePorts=0, ContractBlockType=ContractValidatorBlock, createInportsCheckbox=off}
      mask prompts: assumePorts "Assume ports     :"; guaranteePorts "Guarantee ports :"; modePorts "Mode ports        :"; createInportsCheckbox "Create inports and connect them automatically"
      mask init:
      | set_param(gcb,'LinkStatus','none');
      | contract_callback('inputs_callback',gcb);
      mask DialogControl DescTextVar Prompt: The validator block implements the following logic: <br> <br> <b>Sofar</b>(assume<sub>1</sub> <b>&#8743;</b> assume<sub>2</sub> <b>&#8743;</b> ... assume<sub>k</sub>) <b>&rarr;</b> (guarantee<sub>1</sub> <b>&#8743;</b> guarantee<sub>2</sub> <b>&#8743;</b> ... guarantee<sub>m</sub> <b>&#8743;</b>  mode<sub>1</sub> <b>&#8743;</b> mode<sub>2</sub> <b>&#8743;</b> ... <b>&#8743;</b> mode<sub>n</sub> )<br> where mode<sub>i</sub> = require<sub>i</sub> <b>&rarr;</b> ensure<sub>i</sub>
      mask Display:
      | color('black');
      | port_label('input',1,'assume');
      | port_label('input',2,'guarantee');
      | port_label('output',1,'valid');
  valid : Outport
  wires:
  validator/1 -> valid/1
  code/1 -> guarantee code > -5/4(code)
  PressedDigits/1 -> guarantee code > -5/1(PressedDigits)
  Press/1 -> guarantee code > -5/2(Press)
  Digit/1 -> guarantee code > -5/3(Digit), assume 0 <= Digit and Digit <= 9/1(Digit)
  assume 0 <= Digit and Digit <= 9/1(assume) -> validator/1
  guarantee code > -5/1(guarantee) -> validator/2

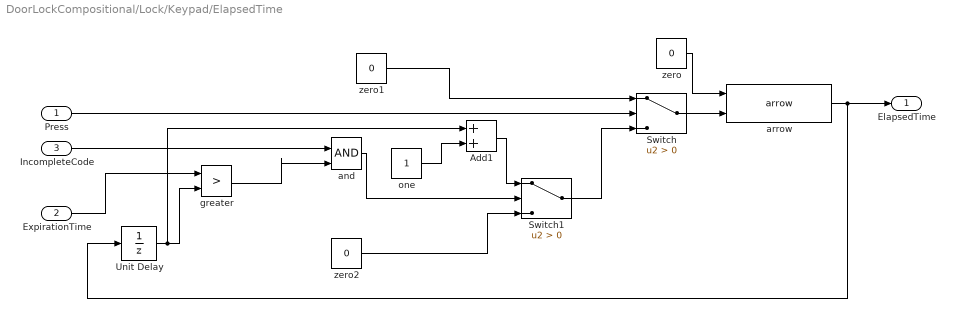
== system DoorLockCompositional/Lock/Keypad/ElapsedTime ==
  Press : Inport  OutDataTypeStr=boolean
  ExpirationTime : Inport  Port=2  OutDataTypeStr=int32
  IncompleteCode : Inport  Port=3  OutDataTypeStr=boolean
  Add1 : Sum  AccumDataTypeStr=int32
  Switch : Switch  Criteria=u2 > Threshold
  Switch1 : Switch  Criteria=u2 > Threshold
  Unit Delay : UnitDelay  SampleTime=-1
  and : Logic  IconShape=distinctive  AllPortsSameDT=off  OutDataTypeStr=boolean
  arrow : Kind/arrow  LustreOperatorBlock=ArrowOperator
  greater : RelationalOperator  Operator=>  OutDataTypeStr=boolean  RndMeth=Nearest
  one : Constant  OutDataTypeStr=int32
  zero : Constant  Value=0  OutDataTypeStr=int32
  zero1 : Constant  Value=0  OutDataTypeStr=int32
  zero2 : Constant  Value=0  OutDataTypeStr=int32
  ElapsedTime : Outport  OutDataTypeStr=int32
  wires:
  zero/1 -> arrow/1
  Press/1 -> Switch/2
  zero1/1 -> Switch/1
  zero2/1 -> Switch1/3
  arrow/1 -> Unit Delay/1, ElapsedTime/1
  Unit Delay/1 -> greater/2, Add1/1
  ExpirationTime/1 -> greater/1
  IncompleteCode/1 -> and/1
  and/1 -> Switch1/2
  greater/1 -> and/2
  Add1/1 -> Switch1/1
  one/1 -> Add1/2
  Switch/1 -> arrow/2
  Switch1/1 -> Switch/3

== system DoorLockCompositional/Lock/Keypad/IncompleteCode ==
  PressedDigits : Inport  OutDataTypeStr=int32
  Compare To Constant : simulink/Logic and Bit Operations/Compare To Constant  relop=<  const=3.0  OutDataTypeStr=boolean
  Compare To Zero : simulink/Logic and Bit Operations/Compare To Zero  relop=>  OutDataTypeStr=boolean
  arrow : Kind/arrow  LustreOperatorBlock=ArrowOperator
  false : Constant  Value=0  OutDataTypeStr=boolean
  pre PressedDigits : Memory
  zero < pre PressedDigits and pre PressedDigits < 3 : Logic  IconShape=distinctive  AllPortsSameDT=off  OutDataTypeStr=boolean
  IncompleteCode : Outport  OutDataTypeStr=boolean
  wires:
  false/1 -> arrow/1
  Compare To Zero/1 -> zero < pre PressedDigits and pre PressedDigits < 3/1
  zero < pre PressedDigits and pre PressedDigits < 3/1 -> arrow/2
  Compare To Constant/1 -> zero < pre PressedDigits and pre PressedDigits < 3/2
  PressedDigits/1 -> pre PressedDigits/1
  pre PressedDigits/1 -> Compare To Constant/1, Compare To Zero/1
  arrow/1 -> IncompleteCode/1

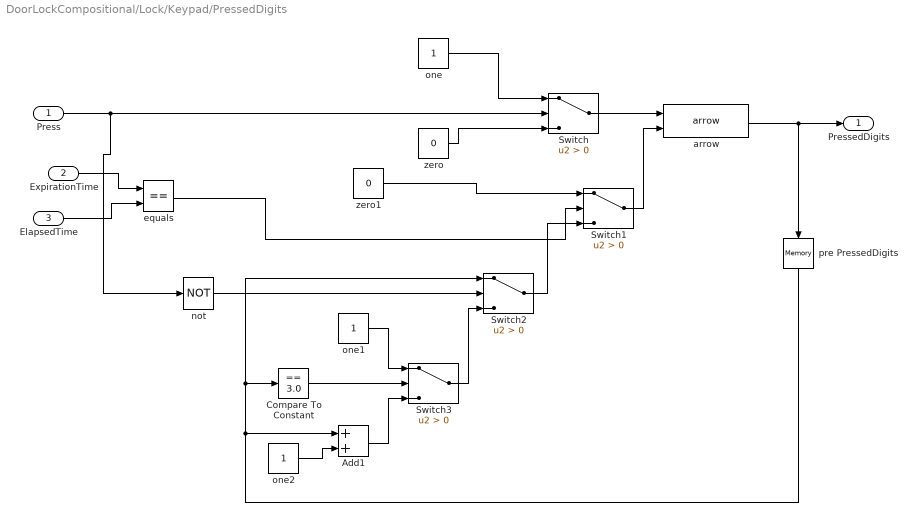
== system DoorLockCompositional/Lock/Keypad/PressedDigits ==
  Press : Inport  OutDataTypeStr=boolean
  ExpirationTime : Inport  Port=2  OutDataTypeStr=int32
  ElapsedTime : Inport  Port=3  OutDataTypeStr=int32
  Add1 : Sum
  Compare To Constant : simulink/Logic and Bit Operations/Compare To Constant  relop===  const=3.0  OutDataTypeStr=boolean
  Switch{,1..3} (4 alike) : Switch  Criteria=u2 > Threshold
  arrow : Kind/arrow  LustreOperatorBlock=ArrowOperator
  equals : RelationalOperator  Operator===  OutDataTypeStr=boolean  RndMeth=Nearest
  not : Logic  Operator=NOT  IconShape=distinctive  AllPortsSameDT=off  OutDataTypeStr=boolean
  one : Constant  OutDataTypeStr=int32
  one1 : Constant  OutDataTypeStr=int32
  one2 : Constant  OutDataTypeStr=int32
  pre PressedDigits : Memory
  zero : Constant  Value=0  OutDataTypeStr=int32
  zero1 : Constant  Value=0  OutDataTypeStr=int32
  PressedDigits : Outport  OutDataTypeStr=int32
  wires:
  Press/1 -> not/1, Switch/2
  one/1 -> Switch/1
  zero/1 -> Switch/3
  Switch/1 -> arrow/1
  arrow/1 -> pre PressedDigits/1, PressedDigits/1
  ExpirationTime/1 -> equals/1
  ElapsedTime/1 -> equals/2
  zero1/1 -> Switch1/1
  equals/1 -> Switch1/2
  not/1 -> Switch2/2
  pre PressedDigits/1 -> Switch2/1, Compare To Constant/1, Add1/1
  Compare To Constant/1 -> Switch3/2
  one1/1 -> Switch3/1
  Switch3/1 -> Switch2/3
  one2/1 -> Add1/2
  Add1/1 -> Switch3/3
  Switch2/1 -> Switch1/3
  Switch1/1 -> arrow/2

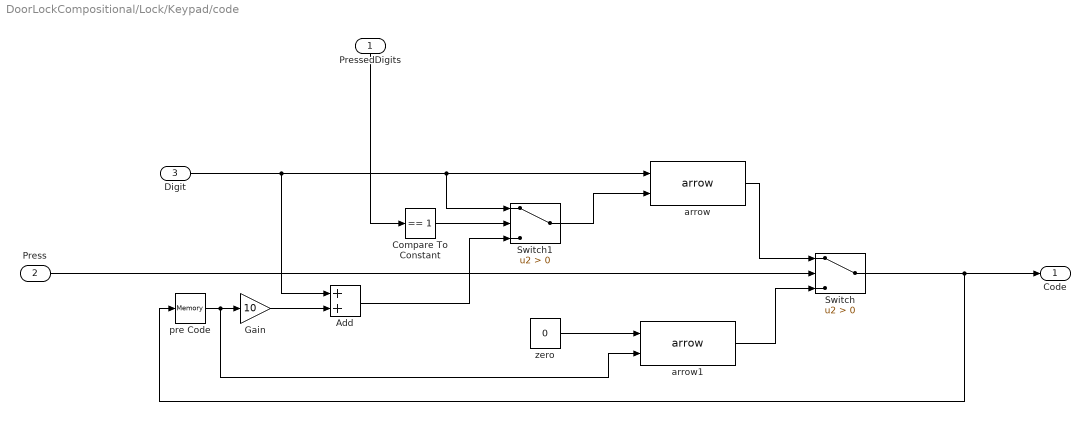
== system DoorLockCompositional/Lock/Keypad/code ==
  PressedDigits : Inport
  Press : Inport  Port=2
  Digit : Inport  Port=3
  Add : Sum  AccumDataTypeStr=int32
  Compare To Constant : simulink/Logic and Bit Operations/Compare To Constant  relop===  const=1  OutDataTypeStr=boolean
  Gain : Gain  Gain=10  OutDataTypeStr=int32
  Switch : Switch  Criteria=u2 > Threshold
  Switch1 : Switch  Criteria=u2 > Threshold
  arrow : Kind/arrow  LustreOperatorBlock=ArrowOperator
  arrow1 : Kind/arrow  LustreOperatorBlock=ArrowOperator
  pre Code : Memory
  zero : Constant  Value=0  OutDataTypeStr=int32
  Code : Outport
  wires:
  arrow1/1 -> Switch/3
  zero/1 -> arrow1/1
  PressedDigits/1 -> Compare To Constant/1
  Digit/1 -> Add/1, Switch1/1, arrow/1
  Press/1 -> Switch/2
  Compare To Constant/1 -> Switch1/2
  Add/1 -> Switch1/3
  pre Code/1 -> arrow1/2, Gain/1
  Gain/1 -> Add/2
  arrow/1 -> Switch/1
  Switch1/1 -> arrow/2
  Switch/1 -> Code/1, pre Code/1

== system DoorLockCompositional/Lock/KeypadSpec/PreRequest ==
  Request : Inport  OutDataTypeStr=boolean
  arrow : Kind/arrow  LustreOperatorBlock=ArrowOperator
  false : Constant  Value=0  OutDataTypeStr=boolean
  pre Request : Memory
  PreRequest : Outport
  wires:
  pre Request/1 -> arrow/2
  arrow/1 -> PreRequest/1
  false/1 -> arrow/1
  Request/1 -> pre Request/1

== system DoorLockCompositional/Lock/KeypadSpec/assume 0 <= Digit and Digit <= 9 ==
  Digit : Inport
  Compare To Constant : simulink/Logic and Bit Operations/Compare To Constant  relop=<=  const=9  OutDataTypeStr=boolean
  Compare To Zero : simulink/Logic and Bit Operations/Compare To Zero  relop=>=  OutDataTypeStr=boolean
  and : Logic  IconShape=distinctive  AllPortsSameDT=off  OutDataTypeStr=boolean
  assume : Outport  OutDataTypeStr=boolean
  wires:
  and/1 -> assume/1
  Digit/1 -> Compare To Constant/1, Compare To Zero/1
  Compare To Zero/1 -> and/1
  Compare To Constant/1 -> and/2

== system DoorLockCompositional/Lock/KeypadSpec/guarantee (not Request) -> (not PreRequest) -> true ==
  Request : Inport
  PreRequest : Inport  Port=2
  first arrow : Kind/arrow  LustreOperatorBlock=ArrowOperator
  not PreRequest : Logic  Operator=NOT  IconShape=distinctive  AllPortsSameDT=off  OutDataTypeStr=boolean
  not Request : Logic  Operator=NOT  IconShape=distinctive  AllPortsSameDT=off  OutDataTypeStr=boolean
  second arrow : Kind/arrow  LustreOperatorBlock=ArrowOperator
  true : Constant  OutDataTypeStr=boolean
  guarantee : Outport  OutDataTypeStr=boolean
  wires:
  Request/1 -> not Request/1
  second arrow/1 -> guarantee/1
  not Request/1 -> first arrow/1
  first arrow/1 -> second arrow/1
  PreRequest/1 -> not PreRequest/1
  not PreRequest/1 -> first arrow/2
  true/1 -> second arrow/2

== system DoorLockCompositional/Lock/KeypadSpec/guarantee Code >= 0 ==
  Code : Inport
  Compare To Zero : simulink/Logic and Bit Operations/Compare To Zero  relop=>=  OutDataTypeStr=boolean
  guarantee : Outport  OutDataTypeStr=boolean
  wires:
  Compare To Zero/1 -> guarantee/1
  Code/1 -> Compare To Zero/1

== system DoorLockCompositional/Lock/KeypadSpec/guarantee Request => (0 <= Code and Code <= 999) ==
  Request : Inport
  Code : Inport  Port=2
  Compare To Constant : simulink/Logic and Bit Operations/Compare To Constant  relop=<=  const=999  OutDataTypeStr=boolean
  Compare To Zero : simulink/Logic and Bit Operations/Compare To Zero  relop=>=  OutDataTypeStr=boolean
  and : Logic  IconShape=distinctive  AllPortsSameDT=off  OutDataTypeStr=boolean
  not Request : Logic  Operator=NOT  IconShape=distinctive  AllPortsSameDT=off  OutDataTypeStr=boolean
  or : Logic  Operator=OR  IconShape=distinctive  AllPortsSameDT=off  OutDataTypeStr=boolean
  guarantee : Outport  OutDataTypeStr=boolean
  wires:
  Code/1 -> Compare To Constant/1, Compare To Zero/1
  and/1 -> or/2
  Compare To Zero/1 -> and/1
  Compare To Constant/1 -> and/2
  Request/1 -> not Request/1
  not Request/1 -> or/1
  or/1 -> guarantee/1

== system DoorLockCompositional/Lock/KeypadSpec/guarantee Request => Press ==
  Press : Inport
  Request : Inport  Port=2
  not Request : Logic  Operator=NOT  IconShape=distinctive  AllPortsSameDT=off  OutDataTypeStr=boolean
  or : Logic  Operator=OR  IconShape=distinctive  AllPortsSameDT=off  OutDataTypeStr=boolean
  guarantee : Outport  OutDataTypeStr=boolean
  wires:
  not Request/1 -> or/1
  Request/1 -> not Request/1
  or/1 -> guarantee/1
  Press/1 -> or/2

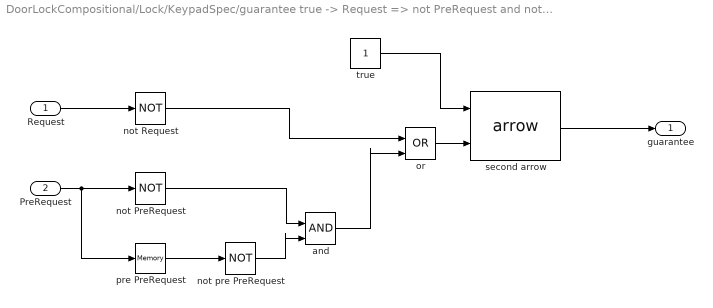
== system DoorLockCompositional/Lock/KeypadSpec/guarantee true -> Request => not PreRequest and not pre PreRequest ==
  Request : Inport
  PreRequest : Inport  Port=2
  and : Logic  IconShape=distinctive  AllPortsSameDT=off  OutDataTypeStr=boolean
  not PreRequest : Logic  Operator=NOT  IconShape=distinctive  AllPortsSameDT=off  OutDataTypeStr=boolean
  not Request : Logic  Operator=NOT  IconShape=distinctive  AllPortsSameDT=off  OutDataTypeStr=boolean
  not pre PreRequest : Logic  Operator=NOT  IconShape=distinctive  AllPortsSameDT=off  OutDataTypeStr=boolean
  or : Logic  Operator=OR  IconShape=distinctive  AllPortsSameDT=off  OutDataTypeStr=boolean
  pre PreRequest : Memory
  second arrow : Kind/arrow  LustreOperatorBlock=ArrowOperator
  true : Constant  OutDataTypeStr=boolean
  guarantee : Outport  OutDataTypeStr=boolean
  wires:
  second arrow/1 -> guarantee/1
  not Request/1 -> or/1
  Request/1 -> not Request/1
  PreRequest/1 -> pre PreRequest/1, not PreRequest/1
  true/1 -> second arrow/1
  pre PreRequest/1 -> not pre PreRequest/1
  not pre PreRequest/1 -> and/2
  not PreRequest/1 -> and/1
  and/1 -> or/2
  or/1 -> second arrow/2

== system DoorLockCompositional/LockSpec/guarantee Since(Locks, not Press) => not Unlocking/Since ==
  X : Inport  OutDataTypeStr=boolean
  Y : Inport  Port=2  OutDataTypeStr=boolean
  and : Logic  IconShape=distinctive  AllPortsSameDT=off  OutDataTypeStr=boolean
  arrow : Kind/arrow  LustreOperatorBlock=ArrowOperator
  false : Constant  Value=0  OutDataTypeStr=boolean
  or : Logic  Operator=OR  IconShape=distinctive  AllPortsSameDT=off  OutDataTypeStr=boolean
  pre SinceXY : Memory
  SinceXY : Outport
  wires:
  X/1 -> or/1
  or/1 -> pre SinceXY/1, SinceXY/1
  Y/1 -> and/1
  false/1 -> arrow/1
  pre SinceXY/1 -> arrow/2
  arrow/1 -> and/2
  and/1 -> or/2

== system DoorLockCompositional/Lock/Keypad/CodeSpec/assume 0 <= Digit and Digit <= 9 ==
  Digit : Inport
  Compare To Constant : simulink/Logic and Bit Operations/Compare To Constant  relop=<=  const=9  OutDataTypeStr=boolean
  Compare To Zero : simulink/Logic and Bit Operations/Compare To Zero  relop=>=  OutDataTypeStr=boolean
  and : Logic  IconShape=distinctive  AllPortsSameDT=off  OutDataTypeStr=boolean
  assume : Outport  OutDataTypeStr=boolean
  wires:
  and/1 -> assume/1
  Digit/1 -> Compare To Constant/1, Compare To Zero/1
  Compare To Zero/1 -> and/1
  Compare To Constant/1 -> and/2

== system DoorLockCompositional/Lock/Keypad/CodeSpec/guarantee code > -5 ==
  PressedDigits : Inport
  Press : Inport  Port=2
  Digit : Inport  Port=3
  code : Inport  Port=4
  Compare To Constant : simulink/Logic and Bit Operations/Compare To Constant  relop=>=  const=-5  OutDataTypeStr=boolean
  Terminator : Terminator
  Terminator1 : Terminator
  Terminator2 : Terminator
  guarantee : Outport  OutDataTypeStr=boolean
  wires:
  code/1 -> Compare To Constant/1
  Compare To Constant/1 -> guarantee/1
  PressedDigits/1 -> Terminator/1
  Press/1 -> Terminator1/1
  Digit/1 -> Terminator2/1
